simulink library "InterModuleProtocol"  (R2020b)
settings: Solver=VariableStepAuto  StartTime=0.0  StopTime=10.0  RelTol=1e-3
(part 1 of 2)
settings Model: Creator=Scythe  LastModifiedBy=Scythe
settings DataIOCC: ReturnWorkspaceOutputs=off
settings DebuggingCC: ArithmeticOperatorsInVariantConditions=warning
settings SFSimCC: CustomCodeUndefinedFunction=UseInterfaceOnly

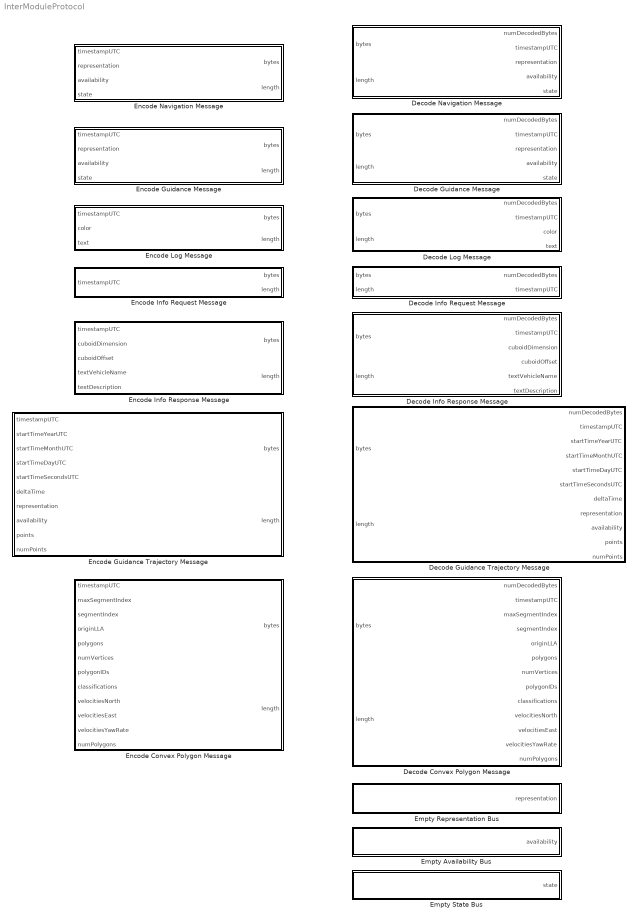
== system InterModuleProtocol ==
  Decode Convex Polygon Message : Subsystem  mask{maxNumPolygons=10}
      mask prompts: maxNumPolygons "Maximum number of polygons:"
      mask help:
      | Decode a convex polygon message (Inter-Module Protocol).<br><br>
      |
      | <b>numDecodedBytes</b><br>Number of decoded bytes (negative value if error occurred).<br><br>
      | <b>timestampUTC</b><br>UTC second of the day.<br><br>
      | <b>maxSegmentIndex</b><br>The maximum segment index number. That is the maximum number of polgon messages belonging to a polygon dataset is (maxSegmentIndex + 1).<br><br>
      | <b>segmentIndex</b><br>The current segment index number for this message.<br><br>
      | <b>originLLA</b><br>Latitude [rad], longitude [rad] and altitude [m] of the origin.<br><br>
      | <b>polygons</b><br>A 2-by-255-by-np matrix containing the vertices for all polygons (column-major order) with np being the maximum number of polygons. A vertex consists of two elements (x and y).<br><br>
      | <b>numVertices</b><br>An np-by-1 vector containing the unique IDs for all polygons in the polygon matrix.<br><br>
      | <b>polygonIDs</b><br>An np-by-1 vector containing the unique IDs for all polygons in the polygon matrix with np being the maximum number of polygons.<br><br>
      | <b>classifications</b><br>An np-by-1 vector containing the classifications for all polygons in the polygon matrix with np being the maximum number of polygons.<br><br>
      | <b>velocitiesNorth</b><br>An np-by-1 vector containing the north velocities in meters per second for all polygons in the polygon matrix with np being the maximum number of polygons.<br><br>
      | <b>velocitiesEast</b><br>An np-by-1 vector containing the east velocities in meters per second for all polygons in the polygon matrix with np being the maximum number of polygons.<br><br>
      | <b>velocitiesYawRate</b><br>An np-by-1 vector containing the rotational rates of turn in radians per second for all polygons in the polygon matrix with np being the maximum number of polygons.<br><br>
      | <b>numPolygons</b><br>The number of decoded polygons.
      mask DialogControl DescGroupVar Prompt: Decode Convex Polygon Message
      mask Display: disp('Decode Convex Polygon Message');
  Decode Guidance Message : Subsystem
      mask help:
      | Decode a guidance message (Inter-Module Protocol).<br><br>
      |
      | <b>numDecodedBytes</b><br>Number of decoded bytes (negative value if error occurred).<br><br>
      | <b>timestampUTC</b><br>UTC second of the day.<br><br>
      | <b>representation</b><br>Representation for the state (0: 4 byte, 1: 8 byte).
      | <br><br>
      |
      | <b>availability</b><br>Availability flags for the state (0: not available, 1: availabe (z), 2: available (xy), 3: available(xyz)).
      | <br><br>
      |
      | <b>state</b><br>State bus.
      mask DialogControl DescGroupVar Prompt: Decode Guidance Message
      mask Display: disp('Decode Guidance Message');
  Decode Guidance Trajectory Message : Subsystem  mask{maxNumPoints=10}
      mask prompts: maxNumPoints "Maximum number of points:"
      mask help:
      | Decode a guidance trajectory message (Inter-Module Protocol).<br><br>
      |
      | <b>numDecodedBytes</b><br>Number of decoded bytes (negative value if error occurred).<br><br>
      | <b>timestampUTC</b><br>UTC second of the day.<br><br>
      | <b>startTimeYearUTC</b><br>Start time for the trajectory: year (UTC).<br><br>
      | <b>startTimeMonthUTC</b><br>Start time for the trajectory: month (UTC), range [1, 12].<br><br>
      | <b>startTimeDayUTC</b><br>Start time for the trajectory: day (UTC), range [1, 31].<br><br>
      | <b>startTimeSecondsUTC</b><br>Start time for the trajectory: seconds of the day (UTC).<br><br>
      | <b>deltaTime</b><br>Time difference from one state point to another in seconds. If this value is set to zero, then each point indicates a waypoint.<br><br>
      | <b>representation</b><br>Representation for all state vectors in the matrix (0: 4 byte, 1: 8 byte).<br><br>
      | <b>availability</b><br>Availability flags for all state vectors in the matrix (0: not available, 1: availabe (z), 2: available (xy), 3: available(xyz)).<br><br>
      | <b>points</b><br>32-by-N matrix containing N state vectors. N is the maximum number of points. Each column of the matrix is as follows:
      | <br>[0]: positionLatitude (rad)
      | <br>[1]: positionLongitude (rad)
      | <br>[2]: positionAltitude (m)
      | <br>[3]: positionNorth (m)
      | <br>[4]: positionEast (m)
      | <br>[5]: positionDown (m)
      | <br>[6]: orientationQuaternionW
      | <br>[7]: orientationQuaternionX
      | <br>[8]: orientationQuaternionY
      | <br>[9]: orientationQuaternionZ
      | <br>[10]: orientationRoll (rad)
      | <br>[11]: orientationPitch (rad)
      | <br>[12]: orientationYaw (rad)
      | <br>[13]: velocityNorth (m/s)
      | <br>[14]: velocityEast (m/s)
      | <br>[15]: velocityDown (m/s)
      | <br>[16]: velocityU (m/s)
      | <br>[17]: velocityV (m/s)
      | <br>[18]: velocityW (m/s)
      | <br>[19]: velocityP (rad/s)
      | <br>[20]: velocityQ (rad/s)
      | <br>[21]: velocityR (rad/s)
      | <br>[22]: accelerationNorth (m/(s*s))
      | <br>[23]: accelerationEast (m/(s*s))
      | <br>[24]: accelerationDown (m/(s*s))
      | <br>[25]: accelerationX (m/(s*s))
      | <br>[26]: accelerationY (m/(s*s))
      | <br>[27]: accelerationZ (m/(s*s))
      | <br>[28]: courseOverGround (rad)
      | <br>[29]: speedOverGround (m/s)
      | <br>[30]: angleOfAttack (rad)
      | <br>[31]: sideSlipAngle (rad)
      | <br><br>
      | <b>numPoints</b><br>Actual number of decoded points inside the output matrix.
      mask DialogControl DescGroupVar Prompt: Decode Guidance Trajectory Message
      mask Display: disp('Decode Guidance Trajectory Message');
  Decode Info Request Message : Subsystem
      mask help:
      | Decode an info request message (Inter-Module Protocol).<br><br>
      |
      | <b>numDecodedBytes</b><br>Number of decoded bytes (negative value if error occurred).<br><br>
      | <b>timestampUTC</b><br>UTC second of the day.
      mask DialogControl DescGroupVar Prompt: Decode Info Request Message
      mask Display: disp('Decode Info Request Message');
  Decode Info Response Message : Subsystem  mask{maxTextLength=255}
      mask prompts: maxTextLength "Maximum output text length (for both textVehicleName and textDescription):"
      mask help:
      | Decode an info response message (Inter-Module Protocol).<br><br>
      |
      | <b>numDecodedBytes</b><br>Number of decoded bytes (negative value if error occurred).<br><br>
      | <b>timestampUTC</b><br>UTC second of the day.<br><br>
      | <b>cuboidDimension</b><br>3-by-1 vector: dimension of the default vehicle cuboid in meters (body-frame).<br><br>
      | <b>cuboidOffset</b><br>3-by-1 vector: offset from body-frame origin to cuboid in meters (body-frame).<br><br>
      | <b>textVehicleName</b><br>The vehicle name text string.<br><br>
      | <b>textDescription</b><br>The optional description text string.
      mask DialogControl DescGroupVar Prompt: Decode Info Response Message
      mask Display: disp('Decode Info Respose Message');
  Decode Log Message : Subsystem  mask{maxTextLength=255}
      mask prompts: maxTextLength "Maximum output text length:"
      mask help:
      | Decode a log message (Inter-Module Protocol).<br><br>
      |
      | <b>numDecodedBytes</b><br>Number of decoded bytes (negative value if error occurred).<br><br>
      | <b>timestampUTC</b><br>UTC second of the day.<br><br>
      | <b>color</b><br>3-by-1 vector containing the color components (red, green, blue).<br><br>
      | <b>text</b><br>The decoded text string.
      mask DialogControl DescGroupVar Prompt: Decode Log Message
      mask Display: disp('Decode Log Message');
  Decode Navigation Message : Subsystem
      mask help:
      | Decode a navigation message (Inter-Module Protocol).<br><br>
      |
      | <b>numDecodedBytes</b><br>Number of decoded bytes (negative value if error occurred).<br><br>
      | <b>timestampUTC</b><br>UTC second of the day.<br><br>
      | <b>representation</b><br>Representation for the state (0: 4 byte, 1: 8 byte).
      | <br><br>
      |
      | <b>availability</b><br>Availability flags for the state (0: not available, 1: availabe (z), 2: available (xy), 3: available(xyz)).
      | <br><br>
      |
      | <b>state</b><br>State bus.
      mask DialogControl DescGroupVar Prompt: Decode Navigation Message
      mask Display: disp('Decode Navigation Message');
  Empty Availability Bus : Subsystem
      mask help: Create an empty availability bus for the Inter-Module Protocol (IMP). All values inside the bus are zero.
      mask DialogControl DescGroupVar Prompt: Empty Availability Bus
      mask Display: disp('Empty Availability Bus\n(IMP)');
  Empty Representation Bus : Subsystem
      mask help: Create an empty representation bus for the Inter-Module Protocol (IMP). All values inside the bus are zero.
      mask DialogControl DescGroupVar Prompt: Empty Representation Bus
      mask Display: disp('Empty Representation Bus\n(IMP)');
  Empty State Bus : Subsystem
      mask help: Create an empty state bus for the Inter-Module Protocol (IMP). All values inside the bus are zero.
      mask DialogControl DescGroupVar Prompt: Empty State Bus
      mask Display: disp('Empty State Bus\n(IMP)');
  Encode Convex Polygon Message : Subsystem  mask{outBufferSize=1024, maxNumPolygons=10}
      mask prompts: outBufferSize "Output buffer size:"; maxNumPolygons "Maximum number of polygons:"
      mask help:
      | Encode a convex polygon message (Inter-Module Protocol).<br><br>
      |
      | <b>timestampUTC</b><br>UTC second of the day.<br><br>
      | <b>maxSegmentIndex</b><br>The maximum segment index number. That is the maximum number of polgon messages belonging to a polygon dataset is (maxSegmentIndex + 1).<br><br>
      | <b>segmentIndex</b><br>The current segment index number for this message.<br><br>
      | <b>originLLA</b><br>Latitude [rad], longitude [rad] and altitude [m] of the origin.<br><br>
      | <b>polygons</b><br>A 2-by-255-by-np matrix containing the vertices for all polygons (column-major order) with np being the maximum number of polygons. A vertex consists of two elements (x and y).<br><br>
      | <b>numVertices</b><br>An np-by-1 vector containing the actual number of vertices per polygon in the polygon matrix.<br><br>
      | <b>polygonIDs</b><br>An np-by-1 vector containing the unique IDs for all polygons in the polygon matrix with np being the maximum number of polygons.<br><br>
      | <b>classifications</b><br>An np-by-1 vector containing the classifications for all polygons in the polygon matrix with np being the maximum number of polygons.<br><br>
      | <b>velocitiesNorth</b><br>An np-by-1 vector containing the north velocities in meters per second for all polygons in the polygon matrix with np being the maximum number of polygons.<br><br>
      | <b>velocitiesEast</b><br>An np-by-1 vector containing the east velocities in meters per second for all polygons in the polygon matrix with np being the maximum number of polygons.<br><br>
      | <b>velocitiesYawRate</b><br>An np-by-1 vector containing the rotational rates of turn in radians per second for all polygons in the polygon matrix with np being the maximum number of polygons.<br><br>
      | <b>numPolygons</b><br>The number of polygons to be used for encoding.
      mask DialogControl DescGroupVar Prompt: Encode Convex Polygon Message
      mask Display: disp('Encode Convex Polygon Message');
  Encode Guidance Message : Subsystem  mask{outputBufferSize=268}
      mask prompts: outputBufferSize "Output buffer size:"
      mask help:
      | Encode a guidance message (Inter-Module Protocol).<br><br>
      |
      | <b>timestampUTC</b><br>UTC second of the day.<br><br>
      | <b>representation</b><br>11-by-1 vector containing the representation for the state (0: 4 byte, 1: 8 byte). Elements indicate:
      | <br>[0]: positionLLA
      | <br>[1]: positionNED
      | <br>[2]: orientationQuaternion
      | <br>[3]: orientationRollPitchYaw
      | <br>[4]: velocityNEDUVW
      | <br>[5]: velocityPQR
      | <br>[6]: accelerationNEDXYZ
      | <br>[7]: courseOverGround
      | <br>[8]: speedOverGround
      | <br>[9]: angleOfAttack
      | <br>[10]: sideSlipAngle
      | <br><br>
      |
      | <b>availability</b><br>13-by-1 vector containing the availability flags for the state (0: not available, 1: availabe (z), 2: available (xy), 3: available(xyz)). Elements indicate:
      | <br>[0]: positionLLA
      | <br>[1]: positionNED
      | <br>[2]: orientationQuaternion (can only be 0 or 1)
      | <br>[3]: orientationRollPitchYaw
      | <br>[4]: velocityNED
      | <br>[5]: velocityUVW
      | <br>[6]: velocityPQR
      | <br>[7]: accelerationNED
      | <br>[8]: accelerationXYZ
      | <br>[9]: courseOverGround (can only be 0 or 1)
      | <br>[10]: speedOverGround (can only be 0 or 1)
      | <br>[11]: angleOfAttack (can only be 0 or 1)
      | <br>[12]: sideSlipAngle (can only be 0 or 1)
      | <br><br>
      |
      | <b>state</b><br>32-by-1 state vector. Elements indicate:
      | <br>[0]: positionLatitude (rad)
      | <br>[1]: positionLongitude (rad)
      | <br>[2]: positionAltitude (m)
      | <br>[3]: positionNorth (m)
      | <br>[4]: positionEast (m)
      | <br>[5]: positionDown (m)
      | <br>[6]: orientationQuaternionW
      | <br>[7]: orientationQuaternionX
      | <br>[8]: orientationQuaternionY
      | <br>[9]: orientationQuaternionZ
      | <br>[10]: orientationRoll (rad)
      | <br>[11]: orientationPitch (rad)
      | <br>[12]: orientationYaw (rad)
      | <br>[13]: velocityNorth (m/s)
      | <br>[14]: velocityEast (m/s)
      | <br>[15]: velocityDown (m/s)
      | <br>[16]: velocityU (m/s)
      | <br>[17]: velocityV (m/s)
      | <br>[18]: velocityW (m/s)
      | <br>[19]: velocityP (rad/s)
      | <br>[20]: velocityQ (rad/s)
      | <br>[21]: velocityR (rad/s)
      | <br>[22]: accelerationNorth (m/(s*s))
      | <br>[23]: accelerationEast (m/(s*s))
      | <br>[24]: accelerationDown (m/(s*s))
      | <br>[25]: accelerationX (m/(s*s))
      | <br>[26]: accelerationY (m/(s*s))
      | <br>[27]: accelerationZ (m/(s*s))
      | <br>[28]: courseOverGround (rad)
      | <br>[29]: speedOverGround (m/s)
      | <br>[30]: angleOfAttack (rad)
      | <br>[31]: sideSlipAngle (rad)
      mask DialogControl DescGroupVar Prompt: Encode Guidance Message
      mask DialogControl Container2 Prompt: Parameters
      mask Display: disp('Encode Guidance Message');
  Encode Guidance Trajectory Message : Subsystem  mask{maxNumPoints=10, outputBufferSize=1024}
      mask prompts: maxNumPoints "Maximum number of points:"; outputBufferSize "Output buffer size:"
      mask help:
      | Encode a guidance trajectory message (Inter-Module Protocol).<br><br>
      |
      | <b>timestampUTC</b><br>UTC second of the day.<br><br>
      | <b>startTimeYearUTC</b><br>Start time for the trajectory: year (UTC).<br><br>
      | <b>startTimeMonthUTC</b><br>Start time for the trajectory: month (UTC), range [1, 12].<br><br>
      | <b>startTimeDayUTC</b><br>Start time for the trajectory: day (UTC), range [1, 31].<br><br>
      | <b>startTimeSecondsUTC</b><br>Start time for the trajectory: seconds of the day (UTC).<br><br>
      | <b>deltaTime</b><br>Time difference from one state point to another in seconds. If this value is set to zero, then each point indicates a waypoint.<br><br>
      | <b>representation</b><br>11-by-1 vector containing the representation for all state points (0: 4 byte, 1: 8 byte). Elements indicate:
      | <br>[0]: positionLLA
      | <br>[1]: positionNED
      | <br>[2]: orientationQuaternion
      | <br>[3]: orientationRollPitchYaw
      | <br>[4]: velocityNEDUVW
      | <br>[5]: velocityPQR
      | <br>[6]: accelerationNEDXYZ
      | <br>[7]: courseOverGround
      | <br>[8]: speedOverGround
      | <br>[9]: angleOfAttack
      | <br>[10]: sideSlipAngle
      | <br><br>
      |
      | <b>availability</b><br>13-by-1 vector containing the availability flags for all state points (0: not available, 1: availabe (z), 2: available (xy), 3: available(xyz)). Elements indicate:
      | <br>[0]: positionLLA
      | <br>[1]: positionNED
      | <br>[2]: orientationQuaternion (can only be 0 or 1)
      | <br>[3]: orientationRollPitchYaw
      | <br>[4]: velocityNED
      | <br>[5]: velocityUVW
      | <br>[6]: velocityPQR
      | <br>[7]: accelerationNED
      | <br>[8]: accelerationXYZ
      | <br>[9]: courseOverGround (can only be 0 or 1)
      | <br>[10]: speedOverGround (can only be 0 or 1)
      | <br>[11]: angleOfAttack (can only be 0 or 1)
      | <br>[12]: sideSlipAngle (can only be 0 or 1)
      | <br><br>
      | <b>points</b><br>32-by-N matrix containing N state vectors. N is the number of points. Each column of the matrix is as follows:
      | <br>[0]: positionLatitude (rad)
      | <br>[1]: positionLongitude (rad)
      | <br>[2]: positionAltitude (m)
      | <br>[3]: positionNorth (m)
      | <br>[4]: positionEast (m)
      | <br>[5]: positionDown (m)
      | <br>[6]: orientationQuaternionW
      | <br>[7]: orientationQuaternionX
      | <br>[8]: orientationQuaternionY
      | <br>[9]: orientationQuaternionZ
      | <br>[10]: orientationRoll (rad)
      | <br>[11]: orientationPitch (rad)
      | <br>[12]: orientationYaw (rad)
      | <br>[13]: velocityNorth (m/s)
      | <br>[14]: velocityEast (m/s)
      | <br>[15]: velocityDown (m/s)
      | <br>[16]: velocityU (m/s)
      | <br>[17]: velocityV (m/s)
      | <br>[18]: velocityW (m/s)
      | <br>[19]: velocityP (rad/s)
      | <br>[20]: velocityQ (rad/s)
      | <br>[21]: velocityR (rad/s)
      | <br>[22]: accelerationNorth (m/(s*s))
      | <br>[23]: accelerationEast (m/(s*s))
      | <br>[24]: accelerationDown (m/(s*s))
      | <br>[25]: accelerationX (m/(s*s))
      | <br>[26]: accelerationY (m/(s*s))
      | <br>[27]: accelerationZ (m/(s*s))
      | <br>[28]: courseOverGround (rad)
      | <br>[29]: speedOverGround (m/s)
      | <br>[30]: angleOfAttack (rad)
      | <br>[31]: sideSlipAngle (rad)
      mask DialogControl DescGroupVar Prompt: Encode Guidance Trajectory Message
      mask Display: disp('Encode Guidance Trajectory Message');
  Encode Info Request Message : Subsystem  mask{outputBufferSize=8}
      mask prompts: outputBufferSize "Output buffer size:"
      mask help:
      | Encode an info request message (Inter-Module Protocol).<br><br>
      |
      | <b>timestampUTC</b><br>UTC second of the day.
      mask DialogControl DescGroupVar Prompt: Encode Info Request Message
      mask DialogControl Container2 Prompt: Parameters
      mask Display: disp('Encode Info Request Message');
  Encode Info Response Message : Subsystem  mask{maxTextLength=255, outputBufferSize=1024}
      mask prompts: maxTextLength "Maximum input text length (for both textVehicleName and textDescription):"; outputBufferSize "Output buffer size:"
      mask help:
      | Encode an info response message (Inter-Module Protocol).<br><br>
      |
      | <b>timestampUTC</b><br>UTC second of the day.<br><br>
      | <b>cuboidDimension</b><br>3-by-1 vector: dimension of the default vehicle cuboid in meters (body-frame).<br><br>
      | <b>cuboidOffset</b><br>3-by-1 vector: offset from body-frame origin to cuboid in meters (body-frame).<br><br>
      | <b>textVehicleName</b><br>The vehicle name text string to be encoded.<br><br>
      | <b>textDescription</b><br>The optional description text string to be encoded.
      mask DialogControl DescGroupVar Prompt: Encode Info Response Message
      mask Display: disp('Encode Info Respose Message');
  Encode Log Message : Subsystem  mask{maxTextLength=255, outputBufferSize=1024}
      mask prompts: maxTextLength "Maximum input text length:"; outputBufferSize "Output buffer size:"
      mask help:
      | Encode a log message (Inter-Module Protocol).<br><br>
      |
      | <b>timestampUTC</b><br>UTC second of the day.<br><br>
      | <b>color</b><br>3-by-1 vector containing the color components (red, green, blue).<br><br>
      | <b>text</b><br>The text string to be encoded.
      mask DialogControl DescGroupVar Prompt: Encode Log Message
      mask Display: disp('Encode Log Message');
  Encode Navigation Message : Subsystem  mask{outputBufferSize=268}
      mask prompts: outputBufferSize "Output buffer size:"
      mask help:
      | Encode a navigation message (Inter-Module Protocol).<br><br>
      |
      | <b>timestampUTC</b><br>UTC second of the day.<br><br>
      | <b>representation</b><br>11-by-1 vector containing the representation for the state (0: 4 byte, 1: 8 byte). Elements indicate:
      | <br>[0]: positionLLA
      | <br>[1]: positionNED
      | <br>[2]: orientationQuaternion
      | <br>[3]: orientationRollPitchYaw
      | <br>[4]: velocityNEDUVW
      | <br>[5]: velocityPQR
      | <br>[6]: accelerationNEDXYZ
      | <br>[7]: courseOverGround
      | <br>[8]: speedOverGround
      | <br>[9]: angleOfAttack
      | <br>[10]: sideSlipAngle
      | <br><br>
      |
      | <b>availability</b><br>13-by-1 vector containing the availability flags for the state (0: not available, 1: availabe (z), 2: available (xy), 3: available(xyz)). Elements indicate:
      | <br>[0]: positionLLA
      | <br>[1]: positionNED
      | <br>[2]: orientationQuaternion (can only be 0 or 1)
      | <br>[3]: orientationRollPitchYaw
      | <br>[4]: velocityNED
      | <br>[5]: velocityUVW
      | <br>[6]: velocityPQR
      | <br>[7]: accelerationNED
      | <br>[8]: accelerationXYZ
      | <br>[9]: courseOverGround (can only be 0 or 1)
      | <br>[10]: speedOverGround (can only be 0 or 1)
      | <br>[11]: angleOfAttack (can only be 0 or 1)
      | <br>[12]: sideSlipAngle (can only be 0 or 1)
      | <br><br>
      |
      | <b>state</b><br>32-by-1 state vector. Elements indicate:
      | <br>[0]: positionLatitude (rad)
      | <br>[1]: positionLongitude (rad)
      | <br>[2]: positionAltitude (m)
      | <br>[3]: positionNorth (m)
      | <br>[4]: positionEast (m)
      | <br>[5]: positionDown (m)
      | <br>[6]: orientationQuaternionW
      | <br>[7]: orientationQuaternionX
      | <br>[8]: orientationQuaternionY
      | <br>[9]: orientationQuaternionZ
      | <br>[10]: orientationRoll (rad)
      | <br>[11]: orientationPitch (rad)
      | <br>[12]: orientationYaw (rad)
      | <br>[13]: velocityNorth (m/s)
      | <br>[14]: velocityEast (m/s)
      | <br>[15]: velocityDown (m/s)
      | <br>[16]: velocityU (m/s)
      | <br>[17]: velocityV (m/s)
      | <br>[18]: velocityW (m/s)
      | <br>[19]: velocityP (rad/s)
      | <br>[20]: velocityQ (rad/s)
      | <br>[21]: velocityR (rad/s)
      | <br>[22]: accelerationNorth (m/(s*s))
      | <br>[23]: accelerationEast (m/(s*s))
      | <br>[24]: accelerationDown (m/(s*s))
      | <br>[25]: accelerationX (m/(s*s))
      | <br>[26]: accelerationY (m/(s*s))
      | <br>[27]: accelerationZ (m/(s*s))
      | <br>[28]: courseOverGround (rad)
      | <br>[29]: speedOverGround (m/s)
      | <br>[30]: angleOfAttack (rad)
      | <br>[31]: sideSlipAngle (rad)
      mask DialogControl DescGroupVar Prompt: Encode Navigation Message
      mask DialogControl Container2 Prompt: Parameters
      mask Display: disp('Encode Navigation Message');

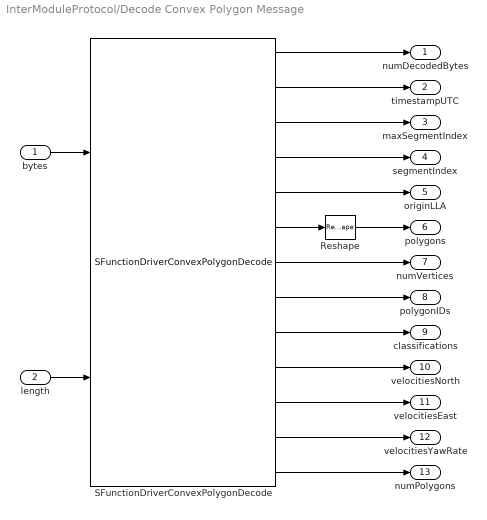
== system InterModuleProtocol/Decode Convex Polygon Message ==
  bytes : Inport  OutDataTypeStr=uint8
  length : Inport  Port=2  OutDataTypeStr=uint32  PortDimensions=1
  Reshape : Reshape  OutputDimensionality=Customize  OutputDimensions=[2,255,maxNumPolygons]
  SFunctionDriverConvexPolygonDecode : S-Function  FunctionName=SFunctionDriverConvexPolygonDecode  Parameters=SParameter1, SampleTime  SFunctionDeploymentMode=off  EnableBusSupport=off  mask(Legacy Function){SFunctionSpec=void OutputDriverConvexPolygonDecode(uint8 u1[], uint32 u2, int32 y1[1], double y2[1], uint8 y3[1], uint8 y4[1], double y5[3], double y6[2*255*p1], uint16 p1, uint8 y7[p1], uint8 y8[p1], uint8 y9[p1], double y10[p1], double y11[p1], double y12[p1], uint16 y13[1]), SParameter1=uint16(reshape(maxNumPolygons, [1 1])), SampleTime=-1, ShowSpec=off}
      mask prompts: SParameter1 "P1:"; SampleTime "Sample time (-1 for inherited):"; ShowSpec "Display function specification"
      mask help:
      | This block allows you to call the legacy functions specified by the following Legacy Code Tool definition:
      | def.SFunctionName = 'SFunctionDriverConvexPolygonDecode';
      | def.OutputFcnSpec = 'void OutputDriverConvexPolygonDecode(uint8 u1[], uint32 u2, int32 y1[1], double y2[1], uint8 y3[1], uint8 y4[1], double y5[3], double y6[2*255*p1], uint16 p1, uint8 y7[p1], uint8 y8[p1], uint8 y9[p1], double y10[p1], double y11[p1], double y12[p1], uint16 y13[1])';
      | def.StartFcnSpec = 'void CreateDriverConvexPolygonDecode()';
      | def.TerminateFcnSpec = 'void DeleteDriverConvexPolygonDecode()';
      | def.HeaderFiles = {'DriverConvexPolygonDecode.h'};
      | def.SourceFiles = {'DriverConvexPolygonDecode.cpp', 'InterModuleProtocol.cpp', 'IMPState.cpp', 'IMPConvexPolygon.cpp', 'IMPStateConfiguration.cpp'};
      | def.SampleTime = 'parameterized';
      | def.Options.useTlcWithAccel = false;
      mask Help: <p>This block was generated automatically by the Legacy Code Tool. For detailed help on this tool, call<a href="matlab:legacy_code('help')"> legacy_code('help')</a>.</p>
      mask Callback ShowSpec:
      | if strcmp(get_param(gcbh, 'ShowSpec'), 'on')
      |   set_param(gcbh, 'MaskDisplay', sprintf('fprintf(''%s'');', get_param(gcbh, 'SFunctionSpec')));
      | else
      |   set_param(gcbh, 'MaskDisplay', sprintf('fprintf(''%s'');', get_param(gcbh, 'FunctionName')));
      | end
      mask Display: fprintf('SFunctionDriverConvexPolygonDecode');
  numDecodedBytes : Outport  OutDataTypeStr=int32  PortDimensions=1  VectorParamsAs1DForOutWhenUnconnected=off
  timestampUTC : Outport  Port=2  OutDataTypeStr=double  Unit=s  PortDimensions=1  VectorParamsAs1DForOutWhenUnconnected=off
  maxSegmentIndex : Outport  Port=3  OutDataTypeStr=uint8  PortDimensions=1  VectorParamsAs1DForOutWhenUnconnected=off
  segmentIndex : Outport  Port=4  OutDataTypeStr=uint8  PortDimensions=1  VectorParamsAs1DForOutWhenUnconnected=off
  originLLA : Outport  Port=5  OutDataTypeStr=double  PortDimensions=3  VectorParamsAs1DForOutWhenUnconnected=off
  polygons : Outport  Port=6  OutDataTypeStr=double  Unit=m  PortDimensions=[2, 255, maxNumPolygons]  VectorParamsAs1DForOutWhenUnconnected=off
  numVertices : Outport  Port=7  OutDataTypeStr=uint8  PortDimensions=maxNumPolygons  VectorParamsAs1DForOutWhenUnconnected=off
  polygonIDs : Outport  Port=8  OutDataTypeStr=uint16  PortDimensions=maxNumPolygons  VectorParamsAs1DForOutWhenUnconnected=off
  classifications : Outport  Port=9  OutDataTypeStr=uint8  PortDimensions=maxNumPolygons  VectorParamsAs1DForOutWhenUnconnected=off
  velocitiesNorth : Outport  Port=10  OutDataTypeStr=double  Unit=m/s  PortDimensions=maxNumPolygons  VectorParamsAs1DForOutWhenUnconnected=off
  velocitiesEast : Outport  Port=11  OutDataTypeStr=double  Unit=m/s  PortDimensions=maxNumPolygons  VectorParamsAs1DForOutWhenUnconnected=off
  velocitiesYawRate : Outport  Port=12  OutDataTypeStr=double  Unit=rad/s  PortDimensions=maxNumPolygons  VectorParamsAs1DForOutWhenUnconnected=off
  numPolygons : Outport  Port=13  OutDataTypeStr=uint16  PortDimensions=1  VectorParamsAs1DForOutWhenUnconnected=off
  wires:
  bytes/1 -> SFunctionDriverConvexPolygonDecode/1
  length/1 -> SFunctionDriverConvexPolygonDecode/2
  Reshape/1 -> polygons/1
  SFunctionDriverConvexPolygonDecode/1 -> numDecodedBytes/1
  SFunctionDriverConvexPolygonDecode/2 -> timestampUTC/1
  SFunctionDriverConvexPolygonDecode/3 -> maxSegmentIndex/1
  SFunctionDriverConvexPolygonDecode/4 -> segmentIndex/1
  SFunctionDriverConvexPolygonDecode/5 -> originLLA/1
  SFunctionDriverConvexPolygonDecode/6 -> Reshape/1
  SFunctionDriverConvexPolygonDecode/7 -> numVertices/1
  SFunctionDriverConvexPolygonDecode/8 -> polygonIDs/1
  SFunctionDriverConvexPolygonDecode/9 -> classifications/1
  SFunctionDriverConvexPolygonDecode/10 -> velocitiesNorth/1
  SFunctionDriverConvexPolygonDecode/11 -> velocitiesEast/1
  SFunctionDriverConvexPolygonDecode/12 -> velocitiesYawRate/1
  SFunctionDriverConvexPolygonDecode/13 -> numPolygons/1

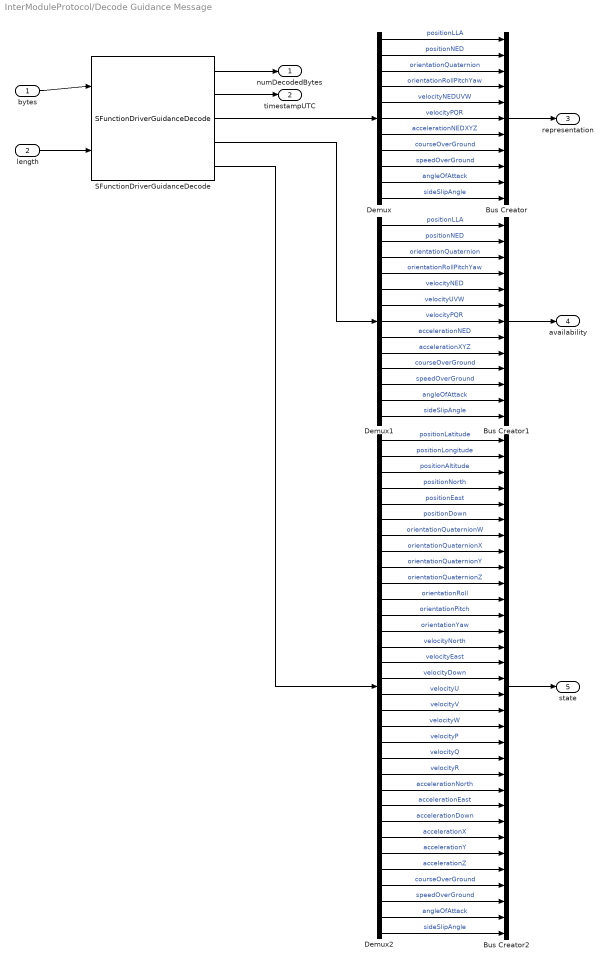
== system InterModuleProtocol/Decode Guidance Message ==
  bytes : Inport  OutDataTypeStr=uint8  PortDimensions=268
  length : Inport  Port=2  OutDataTypeStr=uint32  PortDimensions=1
  Bus Creator : BusCreator  Inputs=11
  Bus Creator1 : BusCreator  Inputs=13
  Bus Creator2 : BusCreator  Inputs=32
  Demux : Demux  Outputs=11
  Demux1 : Demux  Outputs=13
  Demux2 : Demux  Outputs=32
  SFunctionDriverGuidanceDecode : S-Function  FunctionName=SFunctionDriverGuidanceDecode  Parameters=SampleTime  SFunctionDeploymentMode=off  EnableBusSupport=off  mask(Legacy Function){SFunctionSpec=void OutputDriverGuidanceDecode(uint8 u1[], uint32 u2, int32 y1[1], double y2[1], uint8 y3[11], uint8 y4[13], double y5[32]), SampleTime=-1, ShowSpec=off}
      mask prompts: SampleTime "Sample time (-1 for inherited):"; ShowSpec "Display function specification"
      mask help:
      | This block allows you to call the legacy functions specified by the following Legacy Code Tool definition:
      | def.SFunctionName = 'SFunctionDriverGuidanceDecode';
      | def.OutputFcnSpec = 'void OutputDriverGuidanceDecode(uint8 u1[], uint32 u2, int32 y1[1], double y2[1], uint8 y3[11], uint8 y4[13], double y5[32])';
      | def.StartFcnSpec = 'void CreateDriverGuidanceDecode()';
      | def.TerminateFcnSpec = 'void DeleteDriverGuidanceDecode()';
      | def.HeaderFiles = {'DriverGuidanceDecode.h'};
      | def.SourceFiles = {'DriverGuidanceDecode.cpp', 'InterModuleProtocol.cpp', 'IMPState.cpp', 'IMPStateConfiguration.cpp'};
      | def.SampleTime = 'parameterized';
      | def.Options.useTlcWithAccel = false;
      mask Help: <p>This block was generated automatically by the Legacy Code Tool. For detailed help on this tool, call<a href="matlab:legacy_code('help')"> legacy_code('help')</a>.</p>
      mask Callback ShowSpec:
      | if strcmp(get_param(gcbh, 'ShowSpec'), 'on')
      |   set_param(gcbh, 'MaskDisplay', sprintf('fprintf(''%s'');', get_param(gcbh, 'SFunctionSpec')));
      | else
      |   set_param(gcbh, 'MaskDisplay', sprintf('fprintf(''%s'');', get_param(gcbh, 'FunctionName')));
      | end
      mask Display: fprintf('SFunctionDriverGuidanceDecode');
  numDecodedBytes : Outport  OutDataTypeStr=int32  PortDimensions=1  VectorParamsAs1DForOutWhenUnconnected=off
  timestampUTC : Outport  Port=2  OutDataTypeStr=double  Unit=s  PortDimensions=1  VectorParamsAs1DForOutWhenUnconnected=off
  representation : Outport  Port=3  OutDataTypeStr=uint8  PortDimensions=11  VectorParamsAs1DForOutWhenUnconnected=off
  availability : Outport  Port=4  OutDataTypeStr=uint8  PortDimensions=13  VectorParamsAs1DForOutWhenUnconnected=off
  state : Outport  Port=5  OutDataTypeStr=double  PortDimensions=32  VectorParamsAs1DForOutWhenUnconnected=off
  wires:
  length/1 -> SFunctionDriverGuidanceDecode/2
  SFunctionDriverGuidanceDecode/2 -> timestampUTC/1
  bytes/1 -> SFunctionDriverGuidanceDecode/1
  SFunctionDriverGuidanceDecode/1 -> numDecodedBytes/1
  Bus Creator1/1 -> availability/1
  Demux/11 -> Bus Creator/11  "sideSlipAngle"
  Demux/5 -> Bus Creator/5  "velocityNEDUVW"
  Demux/7 -> Bus Creator/7  "accelerationNEDXYZ"
  Demux1/11 -> Bus Creator1/11  "speedOverGround"
  Demux1/10 -> Bus Creator1/10  "courseOverGround"
  Demux1/7 -> Bus Creator1/7  "velocityPQR"
  Demux1/5 -> Bus Creator1/5  "velocityNED"
  Demux1/4 -> Bus Creator1/4  "orientationRollPitchYaw"
  Demux1/6 -> Bus Creator1/6  "velocityUVW"
  Demux/9 -> Bus Creator/9  "speedOverGround"
  SFunctionDriverGuidanceDecode/3 -> Demux/1
  SFunctionDriverGuidanceDecode/4 -> Demux1/1
  Demux1/12 -> Bus Creator1/12  "angleOfAttack"
  Demux/1 -> Bus Creator/1  "positionLLA"
  Demux2/28 -> Bus Creator2/28  "accelerationZ"
  Demux/10 -> Bus Creator/10  "angleOfAttack"
  Bus Creator/1 -> representation/1
  Demux2/29 -> Bus Creator2/29  "courseOverGround"
  Demux1/1 -> Bus Creator1/1  "positionLLA"
  Demux2/30 -> Bus Creator2/30  "speedOverGround"
  Demux1/8 -> Bus Creator1/8  "accelerationNED"
  Demux2/32 -> Bus Creator2/32  "sideSlipAngle"
  Demux2/26 -> Bus Creator2/26  "accelerationX"
  Demux2/24 -> Bus Creator2/24  "accelerationEast"
  Demux1/2 -> Bus Creator1/2  "positionNED"
  Demux2/23 -> Bus Creator2/23  "accelerationNorth"
  Demux1/13 -> Bus Creator1/13  "sideSlipAngle"
  Demux/8 -> Bus Creator/8  "courseOverGround"
  Demux2/27 -> Bus Creator2/27  "accelerationY"
  Demux2/25 -> Bus Creator2/25  "accelerationDown"
  Demux2/21 -> Bus Creator2/21  "velocityQ"
  Demux2/17 -> Bus Creator2/17  "velocityU"
  Demux2/18 -> Bus Creator2/18  "velocityV"
  Demux2/31 -> Bus Creator2/31  "angleOfAttack"
  Demux2/20 -> Bus Creator2/20  "velocityP"
  Demux2/19 -> Bus Creator2/19  "velocityW"
  Demux2/12 -> Bus Creator2/12  "orientationPitch"
  Demux1/3 -> Bus Creator1/3  "orientationQuaternion"
  Demux2/14 -> Bus Creator2/14  "velocityNorth"
  Demux2/10 -> Bus Creator2/10  "orientationQuaternionZ"
  Demux2/13 -> Bus Creator2/13  "orientationYaw"
  Demux1/9 -> Bus Creator1/9  "accelerationXYZ"
  Demux/2 -> Bus Creator/2  "positionNED"
  Demux2/11 -> Bus Creator2/11  "orientationRoll"
  Demux2/16 -> Bus Creator2/16  "velocityDown"
  Demux2/4 -> Bus Creator2/4  "positionNorth"
  Demux2/6 -> Bus Creator2/6  "positionDown"
  Demux/3 -> Bus Creator/3  "orientationQuaternion"
  Demux2/5 -> Bus Creator2/5  "positionEast"
  Demux2/3 -> Bus Creator2/3  "positionAltitude"
  Demux2/7 -> Bus Creator2/7  "orientationQuaternionW"
  Demux2/8 -> Bus Creator2/8  "orientationQuaternionX"
  Demux2/1 -> Bus Creator2/1  "positionLatitude"
  SFunctionDriverGuidanceDecode/5 -> Demux2/1
  Demux2/2 -> Bus Creator2/2  "positionLongitude"
  Demux2/15 -> Bus Creator2/15  "velocityEast"
  Bus Creator2/1 -> state/1
  Demux2/9 -> Bus Creator2/9  "orientationQuaternionY"
  Demux2/22 -> Bus Creator2/22  "velocityR"
  Demux/4 -> Bus Creator/4  "orientationRollPitchYaw"
  Demux/6 -> Bus Creator/6  "velocityPQR"

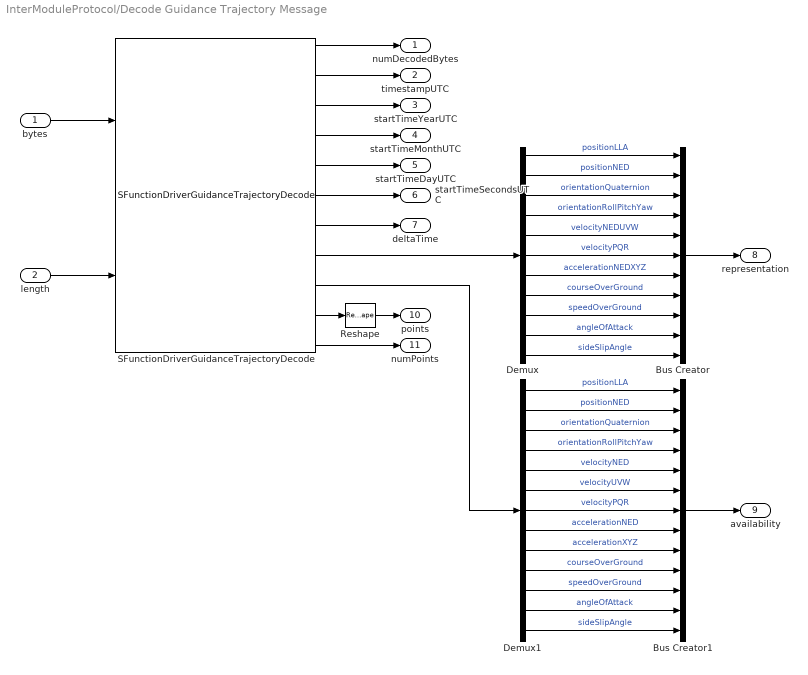
== system InterModuleProtocol/Decode Guidance Trajectory Message ==
  bytes : Inport  OutDataTypeStr=uint8
  length : Inport  Port=2  OutDataTypeStr=uint32  PortDimensions=1
  Bus Creator : BusCreator  Inputs=11
  Bus Creator1 : BusCreator  Inputs=13
  Demux : Demux  Outputs=11
  Demux1 : Demux  Outputs=13
  Reshape : Reshape  OutputDimensionality=Customize  OutputDimensions=[32,maxNumPoints]
  SFunctionDriverGuidanceTrajectoryDecode : S-Function  FunctionName=SFunctionDriverGuidanceTrajectoryDecode  Parameters=SParameter1, SampleTime  SFunctionDeploymentMode=off  EnableBusSupport=off  mask(Legacy Function){SFunctionSpec=void OutputDriverGuidanceTrajectoryDecode(uint8 u1[], uint32 u2, int32 y1[1], double y2[1], int32 y3[1], int32 y4[1], int32 y5[1], double y6[1], double y7[1], uint8 y8[11], uint8 y9[13], double y10[32*p1], uint32 p1, uint32 y11[1]), SParameter1=uint32(reshape(maxNumPoints, [1 1])), SampleTime=-1, ShowSpec=off}
      mask prompts: SParameter1 "P1:"; SampleTime "Sample time (-1 for inherited):"; ShowSpec "Display function specification"
      mask help:
      | This block allows you to call the legacy functions specified by the following Legacy Code Tool definition:
      | def.SFunctionName = 'SFunctionDriverGuidanceTrajectoryDecode';
      | def.OutputFcnSpec = 'void OutputDriverGuidanceTrajectoryDecode(uint8 u1[], uint32 u2, int32 y1[1], double y2[1], int32 y3[1], int32 y4[1], int32 y5[1], double y6[1], double y7[1], uint8 y8[11], uint8 y9[13], double y10[32*p1], uint32 p1, uint32 y11[1])';
      | def.StartFcnSpec = 'void CreateDriverGuidanceTrajectoryDecode()';
      | def.TerminateFcnSpec = 'void DeleteDriverGuidanceTrajectoryDecode()';
      | def.HeaderFiles = {'DriverGuidanceTrajectoryDecode.h'};
      | def.SourceFiles = {'DriverGuidanceTrajectoryDecode.cpp', 'InterModuleProtocol.cpp', 'IMPState.cpp', 'IMPStateConfiguration.cpp'};
      | def.SampleTime = 'parameterized';
      | def.Options.useTlcWithAccel = false;
      mask Help: <p>This block was generated automatically by the Legacy Code Tool. For detailed help on this tool, call<a href="matlab:legacy_code('help')"> legacy_code('help')</a>.</p>
      mask Callback ShowSpec:
      | if strcmp(get_param(gcbh, 'ShowSpec'), 'on')
      |   set_param(gcbh, 'MaskDisplay', sprintf('fprintf(''%s'');', get_param(gcbh, 'SFunctionSpec')));
      | else
      |   set_param(gcbh, 'MaskDisplay', sprintf('fprintf(''%s'');', get_param(gcbh, 'FunctionName')));
      | end
      mask Display: fprintf('SFunctionDriverGuidanceTrajectoryDecode');
  numDecodedBytes : Outport  OutDataTypeStr=int32  PortDimensions=1  VectorParamsAs1DForOutWhenUnconnected=off
  timestampUTC : Outport  Port=2  OutDataTypeStr=double  Unit=s  PortDimensions=1  VectorParamsAs1DForOutWhenUnconnected=off
  startTimeYearUTC : Outport  Port=3  OutDataTypeStr=int32  PortDimensions=1  VectorParamsAs1DForOutWhenUnconnected=off
  startTimeMonthUTC : Outport  Port=4  OutDataTypeStr=int32  PortDimensions=1  VectorParamsAs1DForOutWhenUnconnected=off
  startTimeDayUTC : Outport  Port=5  OutDataTypeStr=int32  PortDimensions=1  VectorParamsAs1DForOutWhenUnconnected=off
  startTimeSecondsUTC : Outport  Port=6  OutDataTypeStr=double  Unit=s  PortDimensions=1  VectorParamsAs1DForOutWhenUnconnected=off
  deltaTime : Outport  Port=7  OutDataTypeStr=double  Unit=s  PortDimensions=1  VectorParamsAs1DForOutWhenUnconnected=off
  representation : Outport  Port=8  VectorParamsAs1DForOutWhenUnconnected=off
  availability : Outport  Port=9  VectorParamsAs1DForOutWhenUnconnected=off
  points : Outport  Port=10  OutDataTypeStr=double  PortDimensions=[32, maxNumPoints]  VectorParamsAs1DForOutWhenUnconnected=off
  numPoints : Outport  Port=11  OutDataTypeStr=uint32  PortDimensions=1  VectorParamsAs1DForOutWhenUnconnected=off
  wires:
  SFunctionDriverGuidanceTrajectoryDecode/5 -> startTimeDayUTC/1
  SFunctionDriverGuidanceTrajectoryDecode/4 -> startTimeMonthUTC/1
  SFunctionDriverGuidanceTrajectoryDecode/2 -> timestampUTC/1
  length/1 -> SFunctionDriverGuidanceTrajectoryDecode/2
  bytes/1 -> SFunctionDriverGuidanceTrajectoryDecode/1
  SFunctionDriverGuidanceTrajectoryDecode/1 -> numDecodedBytes/1
  SFunctionDriverGuidanceTrajectoryDecode/7 -> deltaTime/1
  SFunctionDriverGuidanceTrajectoryDecode/3 -> startTimeYearUTC/1
  SFunctionDriverGuidanceTrajectoryDecode/6 -> startTimeSecondsUTC/1
  Demux/8 -> Bus Creator/8  "courseOverGround"
  Demux1/10 -> Bus Creator1/10  "courseOverGround"
  Demux1/11 -> Bus Creator1/11  "speedOverGround"
  Demux1/13 -> Bus Creator1/13  "sideSlipAngle"
  SFunctionDriverGuidanceTrajectoryDecode/8 -> Demux/1
  Demux1/4 -> Bus Creator1/4  "orientationRollPitchYaw"
  Demux/4 -> Bus Creator/4  "orientationRollPitchYaw"
  SFunctionDriverGuidanceTrajectoryDecode/9 -> Demux1/1
  Demux/9 -> Bus Creator/9  "speedOverGround"
  Demux/3 -> Bus Creator/3  "orientationQuaternion"
  Demux1/6 -> Bus Creator1/6  "velocityUVW"
  Demux1/7 -> Bus Creator1/7  "velocityPQR"
  Demux/2 -> Bus Creator/2  "positionNED"
  Demux1/2 -> Bus Creator1/2  "positionNED"
  Demux/6 -> Bus Creator/6  "velocityPQR"
  Demux1/1 -> Bus Creator1/1  "positionLLA"
  Demux1/9 -> Bus Creator1/9  "accelerationXYZ"
  Bus Creator/1 -> representation/1
  Demux1/3 -> Bus Creator1/3  "orientationQuaternion"
  Demux1/8 -> Bus Creator1/8  "accelerationNED"
  Demux/7 -> Bus Creator/7  "accelerationNEDXYZ"
  Demux/5 -> Bus Creator/5  "velocityNEDUVW"
  Bus Creator1/1 -> availability/1
  Demux/10 -> Bus Creator/10  "angleOfAttack"
  Demux/11 -> Bus Creator/11  "sideSlipAngle"
  Demux1/12 -> Bus Creator1/12  "angleOfAttack"
  Demux/1 -> Bus Creator/1  "positionLLA"
  Demux1/5 -> Bus Creator1/5  "velocityNED"
  Reshape/1 -> points/1
  SFunctionDriverGuidanceTrajectoryDecode/10 -> Reshape/1
  SFunctionDriverGuidanceTrajectoryDecode/11 -> numPoints/1

== system InterModuleProtocol/Decode Info Request Message ==
  bytes : Inport  OutDataTypeStr=uint8  PortDimensions=8
  length : Inport  Port=2  OutDataTypeStr=uint32  PortDimensions=1
  SFunctionDriverInfoRequestDecode : S-Function  FunctionName=SFunctionDriverInfoRequestDecode  Parameters=SampleTime  SFunctionDeploymentMode=off  EnableBusSupport=off  mask(Legacy Function){SFunctionSpec=void OutputDriverInfoRequestDecode(uint8 u1[8], uint32 u2, int32 y1[1], double y2[1]), SampleTime=-1, ShowSpec=on}
      mask prompts: SampleTime "Sample time (-1 for inherited):"; ShowSpec "Display function specification"
      mask help:
      | This block allows you to call the legacy functions specified by the following Legacy Code Tool definition:
      | def.SFunctionName = 'SFunctionDriverInfoRequestDecode';
      | def.OutputFcnSpec = 'void OutputDriverInfoRequestDecode(uint8 u1[8], uint32 u2, int32 y1[1], double y2[1])';
      | def.StartFcnSpec = 'void CreateDriverInfoRequestDecode()';
      | def.TerminateFcnSpec = 'void DeleteDriverInfoRequestDecode()';
      | def.HeaderFiles = {'DriverInfoRequestDecode.h'};
      | def.SourceFiles = {'DriverInfoRequestDecode.cpp', 'InterModuleProtocol.cpp', 'IMPState.cpp', 'IMPStateConfiguration.cpp'};
      | def.SampleTime = 'parameterized';
      | def.Options.useTlcWithAccel = false;
      mask Help: <p>This block was generated automatically by the Legacy Code Tool. For detailed help on this tool, call<a href="matlab:legacy_code('help')"> legacy_code('help')</a>.</p>
      mask Callback ShowSpec:
      | if strcmp(get_param(gcbh, 'ShowSpec'), 'on')
      |   set_param(gcbh, 'MaskDisplay', sprintf('fprintf(''%s'');', get_param(gcbh, 'SFunctionSpec')));
      | else
      |   set_param(gcbh, 'MaskDisplay', sprintf('fprintf(''%s'');', get_param(gcbh, 'FunctionName')));
      | end
      mask Display: fprintf('void OutputDriverInfoRequestDecode(uint8 u1[8], uint32 u2, int32 y1[1], double y2[1])');
  numDecodedBytes : Outport  OutDataTypeStr=int32  PortDimensions=1  VectorParamsAs1DForOutWhenUnconnected=off
  timestampUTC : Outport  Port=2  OutDataTypeStr=double  Unit=s  PortDimensions=1  VectorParamsAs1DForOutWhenUnconnected=off
  wires:
  SFunctionDriverInfoRequestDecode/2 -> timestampUTC/1
  bytes/1 -> SFunctionDriverInfoRequestDecode/1
  length/1 -> SFunctionDriverInfoRequestDecode/2
  SFunctionDriverInfoRequestDecode/1 -> numDecodedBytes/1

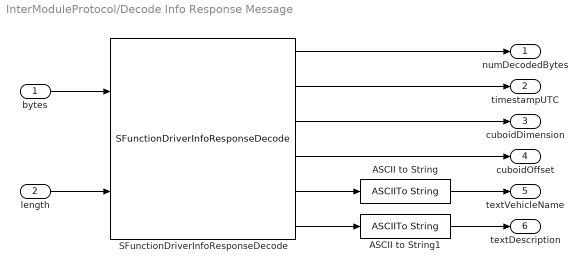
== system InterModuleProtocol/Decode Info Response Message ==
  bytes : Inport  OutDataTypeStr=uint8
  length : Inport  Port=2  OutDataTypeStr=uint32  PortDimensions=1
  ASCII to String : ASCIIToString
  ASCII to String1 : ASCIIToString
  SFunctionDriverInfoResponseDecode : S-Function  FunctionName=SFunctionDriverInfoResponseDecode  Parameters=SParameter1, SampleTime  SFunctionDeploymentMode=off  EnableBusSupport=off  mask(Legacy Function){SFunctionSpec=void OutputDriverInfoResponseDecode(uint8 u1[], uint32 u2, int32 y1[1], double y2[1], double y3[3], double y4[3], uint8 y5[p1], uint8 y6[p1], uint32 p1), SParameter1=uint32(reshape(maxTextLength, [1 1])), SampleTime=-1, ShowSpec=off}
      mask prompts: SParameter1 "P1:"; SampleTime "Sample time (-1 for inherited):"; ShowSpec "Display function specification"
      mask help:
      | This block allows you to call the legacy functions specified by the following Legacy Code Tool definition:
      | def.SFunctionName = 'SFunctionDriverInfoResponseDecode';
      | def.OutputFcnSpec = 'void OutputDriverInfoResponseDecode(uint8 u1[], uint32 u2, int32 y1[1], double y2[1], double y3[3], double y4[3], uint8 y5[p1], uint8 y6[p1], uint32 p1)';
      | def.StartFcnSpec = 'void CreateDriverInfoResponseDecode()';
      | def.TerminateFcnSpec = 'void DeleteDriverInfoResponseDecode()';
      | def.HeaderFiles = {'DriverInfoResponseDecode.h'};
      | def.SourceFiles = {'DriverInfoResponseDecode.cpp', 'InterModuleProtocol.cpp', 'IMPState.cpp', 'IMPStateConfiguration.cpp'};
      | def.SampleTime = 'parameterized';
      | def.Options.useTlcWithAccel = false;
      mask Help: <p>This block was generated automatically by the Legacy Code Tool. For detailed help on this tool, call<a href="matlab:legacy_code('help')"> legacy_code('help')</a>.</p>
      mask Callback ShowSpec:
      | if strcmp(get_param(gcbh, 'ShowSpec'), 'on')
      |   set_param(gcbh, 'MaskDisplay', sprintf('fprintf(''%s'');', get_param(gcbh, 'SFunctionSpec')));
      | else
      |   set_param(gcbh, 'MaskDisplay', sprintf('fprintf(''%s'');', get_param(gcbh, 'FunctionName')));
      | end
      mask Display: fprintf('SFunctionDriverInfoResponseDecode');
  numDecodedBytes : Outport  OutDataTypeStr=int32  PortDimensions=1  VectorParamsAs1DForOutWhenUnconnected=off
  timestampUTC : Outport  Port=2  OutDataTypeStr=double  Unit=s  PortDimensions=1  VectorParamsAs1DForOutWhenUnconnected=off
  cuboidDimension : Outport  Port=3  OutDataTypeStr=double  Unit=m  PortDimensions=3  VectorParamsAs1DForOutWhenUnconnected=off
  cuboidOffset : Outport  Port=4  OutDataTypeStr=double  Unit=m  PortDimensions=3  VectorParamsAs1DForOutWhenUnconnected=off
  textVehicleName : Outport  Port=5  VectorParamsAs1DForOutWhenUnconnected=off
  textDescription : Outport  Port=6  VectorParamsAs1DForOutWhenUnconnected=off
  wires:
  SFunctionDriverInfoResponseDecode/4 -> cuboidOffset/1
  length/1 -> SFunctionDriverInfoResponseDecode/2
  SFunctionDriverInfoResponseDecode/1 -> numDecodedBytes/1
  SFunctionDriverInfoResponseDecode/6 -> ASCII to String1/1
  SFunctionDriverInfoResponseDecode/5 -> ASCII to String/1
  SFunctionDriverInfoResponseDecode/3 -> cuboidDimension/1
  SFunctionDriverInfoResponseDecode/2 -> timestampUTC/1
  bytes/1 -> SFunctionDriverInfoResponseDecode/1
  ASCII to String/1 -> textVehicleName/1
  ASCII to String1/1 -> textDescription/1

== system InterModuleProtocol/Decode Log Message ==
  bytes : Inport
  length : Inport  Port=2
  ASCII to String : ASCIIToString
  SFunctionDriverLogDecode : S-Function  FunctionName=SFunctionDriverLogDecode  Parameters=SParameter1, SampleTime  SFunctionDeploymentMode=off  EnableBusSupport=off  mask(Legacy Function){SFunctionSpec=void OutputDriverLogDecode(uint8 u1[], uint32 u2, int32 y1[1], double y2[1], uint8 y3[3], uint8 y4[p1], uint32 p1), SParameter1=uint32(reshape(maxTextLength, [1 1])), SampleTime=-1, ShowSpec=off}
      mask prompts: SParameter1 "P1:"; SampleTime "Sample time (-1 for inherited):"; ShowSpec "Display function specification"
      mask help:
      | This block allows you to call the legacy functions specified by the following Legacy Code Tool definition:
      | def.SFunctionName = 'SFunctionDriverLogDecode';
      | def.OutputFcnSpec = 'void OutputDriverLogDecode(uint8 u1[], uint32 u2, int32 y1[1], double y2[1], uint8 y3[3], uint8 y4[p1], uint32 p1)';
      | def.StartFcnSpec = 'void CreateDriverLogDecode()';
      | def.TerminateFcnSpec = 'void DeleteDriverLogDecode()';
      | def.HeaderFiles = {'DriverLogDecode.h'};
      | def.SourceFiles = {'DriverLogDecode.cpp', 'InterModuleProtocol.cpp', 'IMPState.cpp', 'IMPStateConfiguration.cpp'};
      | def.SampleTime = 'parameterized';
      | def.Options.useTlcWithAccel = false;
      mask Help: <p>This block was generated automatically by the Legacy Code Tool. For detailed help on this tool, call<a href="matlab:legacy_code('help')"> legacy_code('help')</a>.</p>
      mask Callback ShowSpec:
      | if strcmp(get_param(gcbh, 'ShowSpec'), 'on')
      |   set_param(gcbh, 'MaskDisplay', sprintf('fprintf(''%s'');', get_param(gcbh, 'SFunctionSpec')));
      | else
      |   set_param(gcbh, 'MaskDisplay', sprintf('fprintf(''%s'');', get_param(gcbh, 'FunctionName')));
      | end
      mask Display: fprintf('SFunctionDriverLogDecode');
  numDecodedBytes : Outport  OutDataTypeStr=int32  PortDimensions=1  VectorParamsAs1DForOutWhenUnconnected=off
  timestampUTC : Outport  Port=2  OutDataTypeStr=double  Unit=s  PortDimensions=1  VectorParamsAs1DForOutWhenUnconnected=off
  color : Outport  Port=3  OutDataTypeStr=uint8  PortDimensions=3  VectorParamsAs1DForOutWhenUnconnected=off
  text : Outport  Port=4  VectorParamsAs1DForOutWhenUnconnected=off
  wires:
  SFunctionDriverLogDecode/3 -> color/1
  bytes/1 -> SFunctionDriverLogDecode/1
  SFunctionDriverLogDecode/1 -> numDecodedBytes/1
  length/1 -> SFunctionDriverLogDecode/2
  SFunctionDriverLogDecode/2 -> timestampUTC/1
  SFunctionDriverLogDecode/4 -> ASCII to String/1
  ASCII to String/1 -> text/1
